simulink model "control_sim_discrete"  (R2016b)
settings: Solver=FixedStepAuto  StartTime=0.0  StopTime=10.0  FixedStep=Ts  RelTol=1e-3
values from neighbouring files (symbols this model uses):
  I_wheel = 0.5*m_wheel*r_wheel^2    (= 0.00016224)    [main.m]
  K_d = dlqr(sysd.A,sysd.B,Q,R)    [main.m]
  r_wheel = 104e-3    (= 0.104)    [main.m]
  sysd = c2d(linsys,Ts)    [main.m]
  Ts = 0.01    [main.m]
  z0 = [theta_rad_init; 0; 0; 0]    [main.m]
undefined symbols (not defined in the file or in its folder): DiscIntNeverNeededParam
settings Model: Creator=pluspole  LastModifiedBy=pluspole

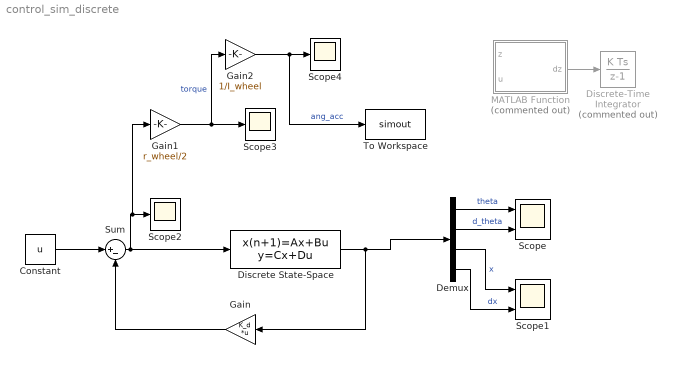
== system control_sim_discrete ==
  Constant : Constant  Value=u  SampleTime=Ts
  Demux : Demux
  Discrete State-Space : DiscreteStateSpace  A=sysd.A  B=sysd.B  C=sysd.C  D=sysd.D  X0=z0  SampleTime=Ts
  Discrete-Time Integrator : DiscreteIntegrator  Commented=on  InitialCondition=z0  InitialConditionSetting=State (most efficient)  SampleTime=Ts  ICPrevOutput=DiscIntNeverNeededParam  ICPrevScaledInput=DiscIntNeverNeededParam
  Gain : Gain  Gain=K_d  Multiplication=Matrix(K*u) (u vector)
  Gain1 : Gain  Gain=r_wheel/2
  Gain2 : Gain  Gain=1/I_wheel
  MATLAB Function : MATLAB Function  Commented=on  TreatAsAtomicUnit=on
  Scope : Scope  NumInputPorts=2
  Scope1 : Scope  NumInputPorts=2
  Scope2 : Scope
  Scope3 : Scope
  Scope4 : Scope
  Sum : Sum  Inputs=|+-
  To Workspace : ToWorkspace  VariableName=simout  SaveFormat=Timeseries  SampleTime=-1
  wires:
  Sum/1 -> Discrete State-Space/1, Gain1/1, Scope2/1
  Gain/1 -> Sum/2
  Constant/1 -> Sum/1
  Demux/1 -> Scope/1  "theta"
  Demux/2 -> Scope/2  "d_theta"
  Demux/3 -> Scope1/1  "x"
  Demux/4 -> Scope1/2  "dx"
  Gain1/1 -> Gain2/1, Scope3/1  "torque"
  Gain2/1 -> To Workspace/1, Scope4/1  "ang_acc"
  MATLAB Function/1(dz) -> Discrete-Time Integrator/1
  Discrete State-Space/1 -> Gain/1, Demux/1

== matlab function control_sim_discrete/MATLAB Function ==
  data: z input; u input; dz output; p parameter
function dz = fcn(z,u, p)

m=p.m;
M=p.M;
l=p.l;
g=p.g;
b=p.b;
k=p.k;

c1=cos(z(1));
s1=sin(z(1));

dz=zeros(4,1);

dz(1,1) = z(2);

dz(2,1) = ((u*c1)-(b*z(3)*c1)-((M+m)*g*s1)+(m*l*c1*s1*(z(2)^2))+((M+m)*((k*z(2))/(l*m))) )/(m*l*(c1^2)-((M+m)*l));
%dy(4,1) = (1/D)*((m+M)*m*g*L*Sy - m*L*Cy*(m*L*y(4)^2*Sy - d*y(2))) - m*L*Cy*(1/D)*u +.01*randn;

dz(3,1) = z(4);

dz(4,1) = (u-(b*z(3))+(m*l*s1*(z(2)^2))-(m*g*c1*s1)+(c1*(k/l)*z(2)))/((M+m)-(m*(c1^2)));
%dy(2,1) = (1/D)*(-m^2*L^2*g*Cy*Sy + m*L^2*(m*L*y(4)^2*Sy - d*y(2))) + m*L*L*(1/D)*u;
